simulink model "lab4Barkalov"  (R2013a)
settings: Solver=ode45  StartTime=0.0  StopTime=10.0  RelTol=1e-3
settings Model: Creator=Ignatiev3  LastModifiedBy=Ignatiev3
settings DataIOCC: SignalLoggingSaveFormat=ModelDataLogs  SignalLoggingName=sigsOut
settings DebuggingCC: SaveWithParameterizedLinksMsg=none  SignalResolutionControl=TryResolveAllWithWarning  SolverPrmCheckMsg=none  MultiTaskDSMMsg=warning  MultiTaskCondExecSysMsg=none  StrictBusMsg=None
settings HardwareCC: TargetUnknown=on
settings RTWCC: IncludeERTFirstTime=on
settings GRTTargetCC: CombineOutputUpdateFcns=off  GRTInterface=on

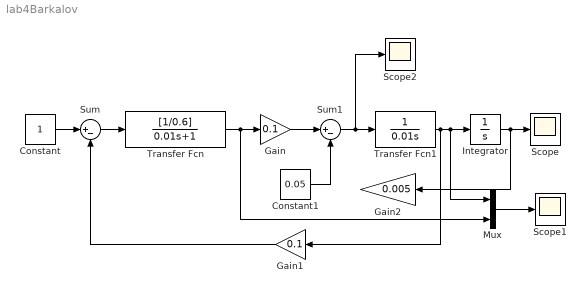
== system lab4Barkalov ==
  Constant : Constant
  Constant1 : Constant  Value=0.05
  Gain : Gain  Gain=0.1  SaturateOnIntegerOverflow=on  OutDataTypeStr=Inherit: Same as input  ParamDataTypeStr=Inherit: Same as input
  Gain1 : Gain  Gain=0.1  SaturateOnIntegerOverflow=on  OutDataTypeStr=Inherit: Same as input  ParamDataTypeStr=Inherit: Same as input
  Gain2 : Gain  Gain=0.005  SaturateOnIntegerOverflow=on  OutDataTypeStr=Inherit: Same as input  ParamDataTypeStr=Inherit: Same as input
  Integrator : Integrator
  Mux : Mux  Inputs=2
  Scope : Scope
      settings: TimeRange=10
  Scope1 : Scope
      settings: TimeRange=10  YMin=-2  YMax=12
  Scope2 : Scope
      settings: SaveName=ScopeData2
  Sum : Sum  Inputs=|+-  SaturateOnIntegerOverflow=on
  Sum1 : Sum  Inputs=|+-  SaturateOnIntegerOverflow=on
  Transfer Fcn : TransferFcn  Numerator=[1/0.6]  Denominator=[0.01 1]
  Transfer Fcn1 : TransferFcn  Denominator=[0.01 0]
  wires:
  Constant/1 -> Sum/1
  Sum/1 -> Transfer Fcn/1
  Gain/1 -> Sum1/1
  Integrator/1 -> Scope/1, Gain2/1
  Gain1/1 -> Sum/2
  Sum1/1 -> Transfer Fcn1/1, Scope2/1
  Transfer Fcn1/1 -> Gain1/1, Mux/1, Integrator/1
  Mux/1 -> Scope1/1
  Transfer Fcn/1 -> Gain/1, Mux/2
  Constant1/1 -> Sum1/2
